simulink model "Copy_of_w13_OOP"  (R2025a)
settings: Solver=VariableStepAuto  StartTime=0.0  StopTime=0.04  FixedStep=1e-5  MaxStep=1e-4  RelTol=1e-3
values from neighbouring files (symbols this model uses):
  B = 0.0001    [main.m]
  J = 0.045    [main.m]
  Kic = Rs*Wcc    (= 1256.63706144)    [main.m]
  Kpc = Lds*Wcc    (= 18.8495559215)    [main.m]
  Lamf = 0.12    [main.m]
  Lds = 30.0e-3    (= 0.03)    [main.m]
  Lqs = 40.0e-3    (= 0.04)    [main.m]
  P = 24    [main.m]
  Rs = 2    [main.m]
  Wcc = 100*2*pi    (= 628.318530718)    [main.m]
libraries: simulink x1
settings Model: Creator=moon  LastModifiedBy=moon
settings RTWCC: GPUComputeCapability=3.5

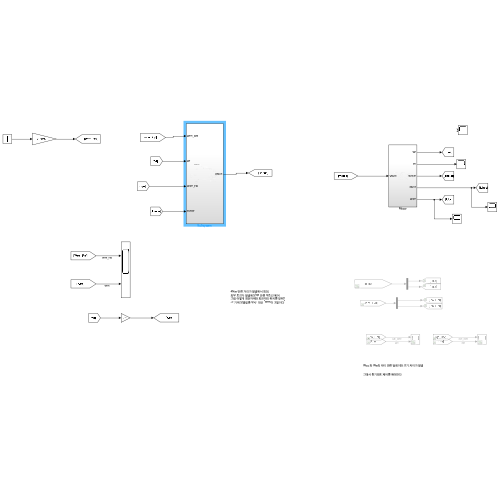
[thumbnail: Simulink's stored preview of the top-level diagram]
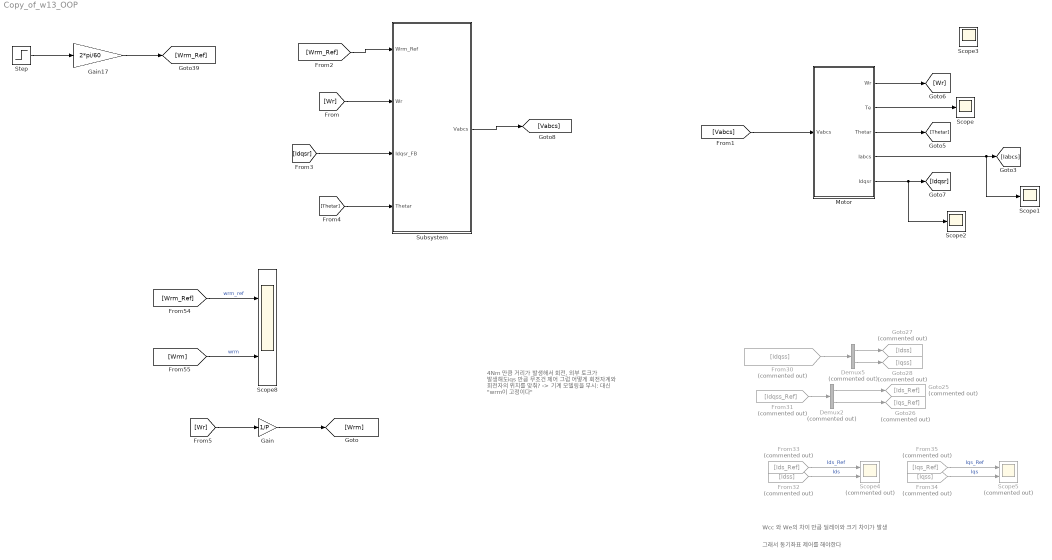
== system Copy_of_w13_OOP ==
  note: 4Nm 만큼 거리가 발생해서 회전,
      | 외부 토크가 발생해도iqs 만큼 무조건 제어
      | 그럼 어떻게 회전자계와 회전자의 위치를 맞춰?
      | -> 기계 모델링을 무시: 대신 "wrm이 고정이다"
  note: 그래서 동기좌표 제어를 해야한다
  note: Wcc 와 We의 차이 만큼 딜레이와 크기 차이가 발생
  Demux2 : Demux  Commented=on  Outputs=2
  Demux5 : Demux  Commented=on  Outputs=2
  From30 : From  Commented=on  GotoTag=Idqss
  From31 : From  Commented=on  GotoTag=Idqss_Ref
  From32 : From  Commented=on  GotoTag=Idss
  From33 : From  Commented=on  GotoTag=Ids_Ref
  From34 : From  Commented=on  GotoTag=Iqss
  From35 : From  Commented=on  GotoTag=Iqs_Ref
  Gain : Gain  Gain=1/P
  Gain17 : Gain  Gain=2*pi/60
  Goto25 : Goto  Commented=on  GotoTag=Ids_Ref
  Goto26 : Goto  Commented=on  GotoTag=Iqs_Ref
  Goto27 : Goto  Commented=on  GotoTag=Idss
  Goto28 : Goto  Commented=on  GotoTag=Iqss
  Motor : Subsystem
  Scope{,1..3} (4 alike) : Scope
      Scope settings: ActiveDisplayYMinimum=-1  ActiveDisplayYMaximum=1  DataLoggingVariableName=ScopeData10
      Scope1 settings: ActiveDisplayYMinimum=-1  ActiveDisplayYMaximum=1  DataLoggingVariableName=ScopeData11
      Scope2 settings: ActiveDisplayYMinimum=-1  ActiveDisplayYMaximum=1  DataLoggingVariableName=ScopeData12
      Scope3 settings: DataLoggingVariableName=ScopeData13
  Scope4 : Scope  Commented=on  NumInputPorts=2
      settings: ActiveDisplayYMinimum=-5.10751  ActiveDisplayYMaximum=5.1663  DataLoggingVariableName=ScopeData2
  Scope5 : Scope  Commented=on  NumInputPorts=2
      settings: ActiveDisplayYMinimum=-5.08231  ActiveDisplayYMaximum=5.15483  DataLoggingVariableName=ScopeData3
  Scope8 : Scope  NumInputPorts=2
      settings: ActiveDisplayYMinimum=-64.34522  ActiveDisplayYMaximum=579.10702
  Step : Step  After=4000  SampleTime=0
  Subsystem : Subsystem
  wires:
  Demux2/2 -> Goto26/1
  Demux2/1 -> Goto25/1
  From31/1 -> Demux2/1
  From30/1 -> Demux5/1
  Demux5/1 -> Goto27/1
  Demux5/2 -> Goto28/1
  From33/1 -> Scope4/1  "Ids_Ref"
  From32/1 -> Scope4/2  "Ids"
  From34/1 -> Scope5/2  "Iqs"
  From35/1 -> Scope5/1  "Iqs_Ref"
  [Wrm_Ref] -> Scope8/1  "wrm_ref"
  [Wrm] -> Scope8/2  "wrm"
  Gain17/1 -> [Wrm_Ref]
  Step/1 -> Gain17/1
  Motor/4(Iabcs) -> Scope1/1, [Iabcs]
  Motor/3(Thetar) -> [Thetar]
  Motor/1(Wr) -> [Wr]
  [Vabcs] -> Motor/1(Vabcs)
  Motor/5(Idqsr) -> Scope2/1, [Idqsr]
  [Wr] -> Subsystem/2(Wr)
  [Idqsr] -> Subsystem/3(Idqsr_FB)
  Subsystem/1(Vabcs) -> [Vabcs]
  [Thetar] -> Subsystem/4(Thetar)
  [Wrm_Ref] -> Subsystem/1(Wrm_Ref)
  [Wr] -> Gain/1
  Gain/1 -> [Wrm]
  Motor/2(Te) -> Scope/1

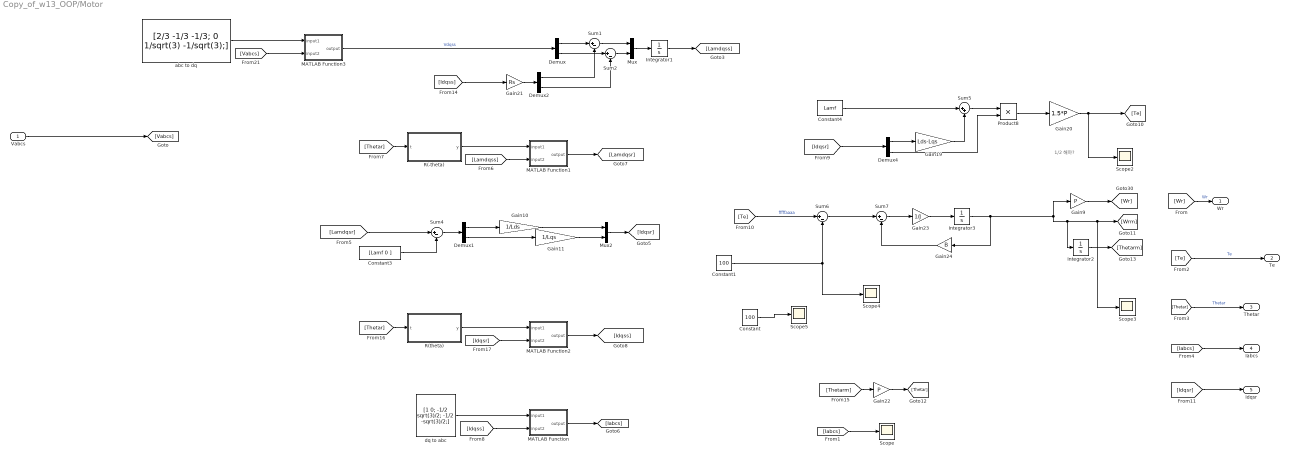
== system Copy_of_w13_OOP/Motor ==
  note: 1/2 해야?
  Vabcs : Inport
  Constant : Constant  Value=100
  Constant1 : Constant  Value=100
  Constant3 : Constant  Value=[Lamf 0 ]
  Constant4 : Constant  Value=Lamf
  Demux{,1..2,4} (4 alike) : Demux  Outputs=2
  Gain10 : Gain  Gain=1/Lds
  Gain11 : Gain  Gain=1/Lqs
  Gain19 : Gain  Gain=Lds-Lqs
  Gain20 : Gain  Gain=1.5*P
  Gain21 : Gain  Gain=Rs
  Gain22 : Gain  Gain=P
  Gain23 : Gain  Gain=1/J
  Gain24 : Gain  Gain=B
  Gain9 : Gain  Gain=P
  Integrator1 : Integrator
  Integrator2 : Integrator
  Integrator3 : Integrator
  MATLAB Function : MATLAB Function  TreatAsAtomicUnit=on
  MATLAB Function1 : MATLAB Function  TreatAsAtomicUnit=on
  MATLAB Function2 : MATLAB Function  TreatAsAtomicUnit=on
  MATLAB Function3 : MATLAB Function  TreatAsAtomicUnit=on
  Mux : Mux  Inputs=2
  Mux2 : Mux  Inputs=2
  Product8 : Product
  R(-theta) : Subsystem
      mask Display: image(imread('img/rotateInverseMatrix.png'))
  R(theta) : Subsystem
      mask Display: image(imread('img/rotateMatrix.png'))
  Scope{,2..5} (5 alike) : Scope
      Scope settings: ActiveDisplayYMinimum=-12.65498  ActiveDisplayYMaximum=12.66704
      Scope2 settings: ActiveDisplayYMinimum=-30.63126  ActiveDisplayYMaximum=63.40805  DataLoggingVariableName=ScopeData2
      Scope3 settings: ActiveDisplayYMinimum=-7240.0541502508459  ActiveDisplayYMaximum=1269.8716380292226  DataLoggingVariableName=ScopeData7
      Scope4 settings: ActiveDisplayYMinimum=-12.499999999999996  ActiveDisplayYMaximum=112.5  DataLoggingVariableName=ScopeData8
      Scope5 settings: ActiveDisplayYMinimum=90  ActiveDisplayYMaximum=110  DataLoggingVariableName=ScopeData9
  Sum{1..2,4,6..7} (5 alike) : Sum  Inputs=|+-
  Sum5 : Sum  Inputs=|++
  abc to dq : Constant  Value=[2/3 -1/3 -1/3; 0 1/sqrt(3) -1/sqrt(3);]
      mask Display: image(imread('img/abc2dq.png'))
  dq to abc : Constant  Value=[1 0; -1/2 sqrt(3)/2; -1/2 -sqrt(3)/2;]
      mask Display: image(imread('img/dq2abc.png'))
  Wr : Outport
  Te : Outport  Port=2
  Thetar : Outport  Port=3
  Iabcs : Outport  Port=4
  Idqsr : Outport  Port=5
  wires:
  R(-theta)/1(y) -> MATLAB Function1/1(input1)
  [Idqsr] -> Demux4/1
  Product8/1 -> Gain20/1
  Sum7/1 -> Gain23/1
  Sum5/1 -> Product8/1
  [Thetar] -> R(theta)/1(t)
  [Lamdqsr] -> Sum4/1
  [Idqss] -> Gain21/1
  R(theta)/1(y) -> MATLAB Function2/1(input1)
  Gain24/1 -> Sum7/2
  MATLAB Function/1(output) -> [Iabcs]
  Constant4/1 -> Sum5/1
  [Thetar] -> R(-theta)/1(t)
  MATLAB Function2/1(output) -> [Idqss]
  [Vabcs] -> MATLAB Function3/2(input2)
  Demux1/2 -> Gain11/1
  abc to dq/1 -> MATLAB Function3/1(input1)
  Gain20/1 -> Scope2/1, [Te]
  Integrator1/1 -> [Lamdqss]
  [Iabcs] -> Scope/1
  [Idqsr] -> MATLAB Function2/2(input2)
  Gain23/1 -> Integrator3/1
  Demux1/1 -> Gain10/1
  [Idqss] -> MATLAB Function/2(input2)
  Gain19/1 -> Sum5/2
  dq to abc/1 -> MATLAB Function/1(input1)
  Gain11/1 -> Mux2/2
  Demux4/2 -> Product8/2
  MATLAB Function1/1(output) -> [Lamdqsr]
  Mux2/1 -> [Idqsr]
  Constant3/1 -> Sum4/2
  Gain10/1 -> Mux2/1
  [Te] -> Sum6/1  "fffffaaaa"
  Gain22/1 -> [Thetar]
  Integrator3/1 -> Gain24/1, Integrator2/1, Scope3/1, [Wrm], Gain9/1
  Integrator2/1 -> [Thetarm]
  Sum6/1 -> Sum7/1
  [Lamdqss] -> MATLAB Function1/2(input2)
  [Thetarm] -> Gain22/1
  Sum4/1 -> Demux1/1
  Demux4/1 -> Gain19/1
  Vabcs/1 -> [Vabcs]
  [Wr] -> Wr/1  "Wr"
  [Te] -> Te/1  "Te"
  [Thetar] -> Thetar/1  "Thetar"
  [Iabcs] -> Iabcs/1
  [Idqsr] -> Idqsr/1
  MATLAB Function3/1(output) -> Demux/1  "Vdqss"
  Gain21/1 -> Demux2/1
  Sum2/1 -> Mux/2
  Sum1/1 -> Mux/1
  Demux2/1 -> Sum1/2
  Demux2/2 -> Sum2/2
  Demux/2 -> Sum2/1
  Demux/1 -> Sum1/1
  Mux/1 -> Integrator1/1
  Constant1/1 -> Sum6/2, Scope4/1
  Gain9/1 -> [Wr]
  Constant/1 -> Scope5/1

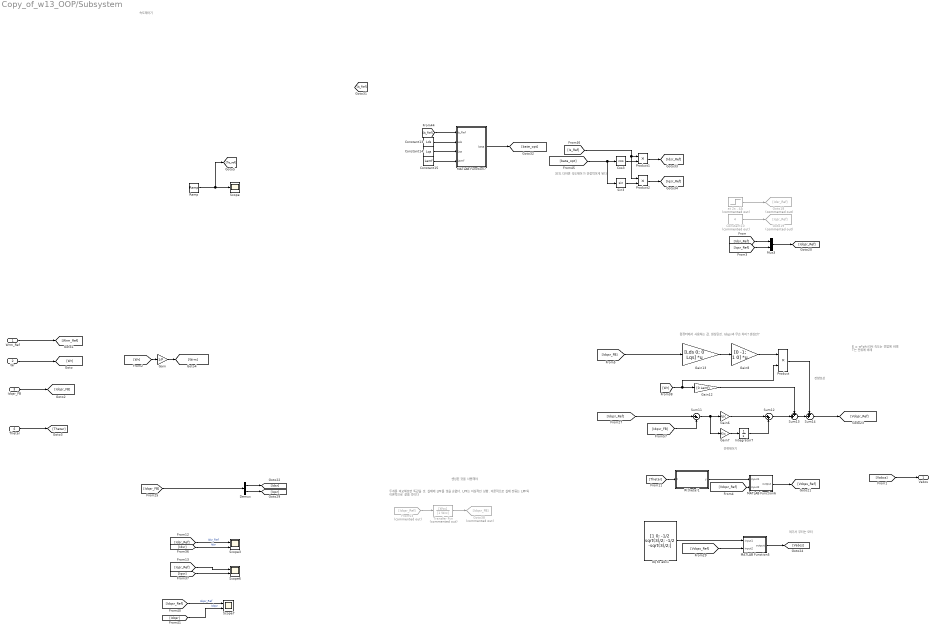
== system Copy_of_w13_OOP/Subsystem ==
  note: 30도 더하면 속도제어가 안정적이게 된다
  note: E = w*phi 라서 속도는 전압에 비례
      | T는 전류에 비례
  note: 전류제어기
  note: 컴퓨터에서 사용하는 값. 센싱된것. Idqsr과 무슨 차이? 센싱만?
  note: 센싱된 것을 사용해야
  note: 여기서 부터는 모터
  note: 두개를 비교해보면 똑같을 것. 실제에 LPF를 넣을 순없다. LPF는 이상적인 상황. 이론적으로 실제 전류는 LPF와 이론적으로 같을 것이다
  note: 속도제어기
  note: 전향보상
  Wrm_Ref : Inport
  Wr : Inport  Port=2
  Idqsr_FB : Inport  Port=3
  Thetar : Inport  Port=4
  Constant10 : Constant  Commented=on  Value=4
  Constant13 : Constant  Value=Lds
  Constant14 : Constant  Value=Lqs
  Constant15 : Constant  Value=Lamf
  Cos3 : Trigonometry  Operator=cos
  Demux : Demux  Outputs=2
  From53 : From  Commented=on  GotoTag=Idqsr_Ref
  Gain : Gain  Gain=1/P
  Gain12 : Gain  Gain=[0 Lamf]
  Gain13 : Gain  Gain=[Lds 0; 0 Lqs]  Multiplication=Matrix(K*u)
  Gain6 : Gain  Gain=Kpc
  Gain7 : Gain  Gain=Kic
  Gain8 : Gain  Gain=[0 -1; 1 0]  Multiplication=Matrix(K*u)
  Goto18 : Goto  Commented=on  GotoTag=Idsr_Ref
  Goto19 : Goto  Commented=on  GotoTag=Iqsr_Ref
  Goto38 : Goto  Commented=on  GotoTag=Idqsr_FB
  Integrator7 : Integrator
  MATLAB Function5 : MATLAB Function  TreatAsAtomicUnit=on
  MATLAB Function6 : MATLAB Function  TreatAsAtomicUnit=on
  MATLAB Function7 : MATLAB Function  TreatAsAtomicUnit=on
  Mux3 : Mux  Inputs=2
  Product : Product
  Product1 : Product
  Product2 : Product
  R(theta)1 : Subsystem
      mask Display: image(imread('img/rotateMatrix.png'))
  Ramp : simulink/Sources/Ramp  slope=100  start=0  InitialOutput=0
  Scope : Scope
      settings: ActiveDisplayYMinimum=-0.0049999999999999992  ActiveDisplayYMaximum=0.045
  Scope3 : Scope  NumInputPorts=2
      settings: ActiveDisplayYMinimum=-5.30172  ActiveDisplayYMaximum=0.86593  DataLoggingVariableName=ScopeData4
  Scope6 : Scope  NumInputPorts=2
      settings: ActiveDisplayYMinimum=-0.50888  ActiveDisplayYMaximum=4.57994  DataLoggingVariableName=ScopeData5
  Scope7 : Scope  NumInputPorts=2
      settings: ActiveDisplayYMinimum=-5.25048  ActiveDisplayYMaximum=7.25433  DataLoggingVariableName=ScopeData6
  Sin3 : Trigonometry
  Sum11 : Sum  Inputs=|+-
  Sum12 : Sum  Inputs=|++
  Sum13 : Sum  Inputs=++|
  Sum14 : Sum  Inputs=++|
  Transfer Fcn : TransferFcn  Commented=on  Numerator=[Wcc]  Denominator=[1 Wcc]
  "at 2s , 4A" : Step  Commented=on  Time=2  After=4  SampleTime=0
  dq to abc1 : Constant  Value=[1 0; -1/2 sqrt(3)/2; -1/2 -sqrt(3)/2;]
      mask Display: image(imread('img/dq2abc.png'))
  Vabcs : Outport
  wires:
  [Vdqss_Ref] -> MATLAB Function5/2(input2)
  Constant14/1 -> MATLAB Function7/3(Lqs)
  Product/1 -> Sum14/1
  Product2/1 -> [Iqsr_Ref]
  Product1/1 -> [Idsr_Ref]
  [Thetar] -> R(theta)1/1(t)
  [Idqsr] -> Scope7/2  "Idqsr"
  Constant13/1 -> MATLAB Function7/2(Lds)
  [Iqsr_Ref] -> Mux3/2
  Transfer Fcn/1 -> Goto38/1
  [Idsr_Ref] -> Mux3/1
  "at 2s , 4A"/1 -> Goto18/1
  [Idqsr_FB] -> Gain13/1
  [Iqsr_Ref] -> Scope6/1
  R(theta)1/1(y) -> MATLAB Function6/1(input1)
  Cos3/1 -> Product1/2
  [Idqsr_Ref] -> Scope7/1  "Idqsr_Ref"
  Demux/2 -> [Iqsr]
  Sin3/1 -> Product2/2
  Gain13/1 -> Gain8/1
  [Idsr] -> Scope3/2  "Idsr"
  [Is_Ref] -> MATLAB Function7/1(Is_Ref)
  MATLAB Function6/1(output) -> [Vdqss_Ref]
  Sum14/1 -> [Vdqsr_Ref]
  Sum13/1 -> Sum14/2
  [bate_opt] -> Sin3/1, Cos3/1
  Constant15/1 -> MATLAB Function7/4(Lamf)
  dq to abc1/1 -> MATLAB Function5/1(input1)
  Constant10/1 -> Goto19/1
  Demux/1 -> [Idsr]
  [Idqsr_FB] -> Sum11/2
  Integrator7/1 -> Sum12/2
  Gain8/1 -> Product/1
  [Idsr_Ref] -> Scope3/1  "Idsr_Ref"
  Gain6/1 -> Sum12/1
  [Wr] -> Product/2, Gain12/1
  [Idqsr_Ref] -> Sum11/1
  [Is_Ref] -> Product2/1, Product1/1
  MATLAB Function7/1(beta) -> [bate_opt]
  MATLAB Function5/1(output) -> [Vabcs]
  [Iqsr] -> Scope6/2
  Mux3/1 -> [Idqsr_Ref]
  Gain12/1 -> Sum13/1
  [Idqsr_FB] -> Demux/1
  Sum11/1 -> Gain7/1, Gain6/1
  [Vdqsr_Ref] -> MATLAB Function6/2(input2)
  Sum12/1 -> Sum13/2
  Gain7/1 -> Integrator7/1
  From53/1 -> Transfer Fcn/1
  Wrm_Ref/1 -> [Wrm_Ref]
  Wr/1 -> [Wr]
  Idqsr_FB/1 -> [Idqsr_FB]
  [Vabcs] -> Vabcs/1
  Thetar/1 -> [Thetar]
  [Wr] -> Gain/1
  Gain/1 -> [Wrm]
  Ramp/1 -> [Te_ref], Scope/1

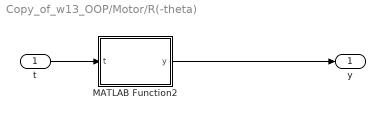
== system Copy_of_w13_OOP/Motor/R(-theta) ==
  t : Inport
  MATLAB Function2 : MATLAB Function  TreatAsAtomicUnit=on
  y : Outport
  wires:
  MATLAB Function2/1(y) -> y/1
  t/1 -> MATLAB Function2/1(t)

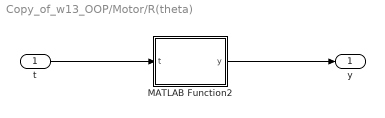
== system Copy_of_w13_OOP/Motor/R(theta) ==
  t : Inport
  MATLAB Function2 : MATLAB Function  TreatAsAtomicUnit=on
  y : Outport
  wires:
  MATLAB Function2/1(y) -> y/1
  t/1 -> MATLAB Function2/1(t)

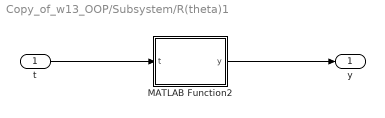
== system Copy_of_w13_OOP/Subsystem/R(theta)1 ==
  t : Inport
  MATLAB Function2 : MATLAB Function  TreatAsAtomicUnit=on
  y : Outport
  wires:
  MATLAB Function2/1(y) -> y/1
  t/1 -> MATLAB Function2/1(t)

== matlab function Copy_of_w13_OOP/Motor/MATLAB Function1 ==
  data: input1 input; output output; input2 input
function output = matrix_multiply(input1, input2)
    % 행렬 곱셈 (input1의 열 수 = input2의 행 수)
    output = input1 * input2;
end

== matlab function Copy_of_w13_OOP/Motor/MATLAB Function ==
  data: input1 input; output output; input2 input
function output = matrix_multiply(input1, input2)
    % 행렬 곱셈 (input1의 열 수 = input2의 행 수)
    output = input1 * input2;
end

== matlab function Copy_of_w13_OOP/Motor/R(-theta)/MATLAB Function2 ==
  data: t input; y output
function y = matrix_output(t)
y = [cos(t) sin(t); -sin(t) cos(t)];

== matlab function Copy_of_w13_OOP/Motor/MATLAB Function2 ==
  data: input1 input; output output; input2 input
function output = matrix_multiply(input1, input2)
    % 행렬 곱셈 (input1의 열 수 = input2의 행 수)
    output = input1 * input2;
end

== matlab function Copy_of_w13_OOP/Motor/R(theta)/MATLAB Function2 ==
  data: t input; y output
function y = matrix_output(t)
y = [cos(t) -sin(t); sin(t) cos(t)];

== matlab function Copy_of_w13_OOP/Motor/MATLAB Function3 ==
  data: input1 input; output output; input2 input
function output = matrix_multiply(input1, input2)
    % 행렬 곱셈 (input1의 열 수 = input2의 행 수)
    output = input1 * input2;
end

== matlab function Copy_of_w13_OOP/Subsystem/MATLAB Function5 ==
  data: input1 input; output output; input2 input
function output = matrix_multiply(input1, input2)
    % 행렬 곱셈 (input1의 열 수 = input2의 행 수)
    output = input1 * input2;
end

== matlab function Copy_of_w13_OOP/Subsystem/MATLAB Function6 ==
  data: input1 input; output output; input2 input
function output = matrix_multiply(input1, input2)
    % 행렬 곱셈 (input1의 열 수 = input2의 행 수)
    output = input1 * input2;
end

== matlab function Copy_of_w13_OOP/Subsystem/R(theta)1/MATLAB Function2 ==
  data: t input; y output
function y = matrix_output(t)
y = [cos(t) -sin(t); sin(t) cos(t)];

== matlab function Copy_of_w13_OOP/Subsystem/MATLAB Function7 ==
  data: Is_Ref input; beta output; Lds input; Lqs input; Lamf input
function beta = fcn(Is_Ref, Lds, Lqs, Lamf)

beta = acos((-Lamf+sqrt(Lamf^2+8*(Lds-Lqs)^2*Is_Ref^2))/(4*(Lds-Lqs)*(Is_Ref+0.001)));
